simulink model "state_space_simulink_feedback_control101"  (R2023b)
settings: Solver=VariableStepAuto  StartTime=0.0  StopTime=endtime  RelTol=1e-3
undefined symbols (not defined in the file or in its folder): A, B, C, Cx, Dx, K, x0
settings Model: Creator=Anthony  LastModifiedBy=Anthony Rossiter
settings DataIOCC: SaveFormat=Structure  SignalLogging=off
settings ModelReferenceCC: EnableRefExpFcnMdlSchedulingChecks=on

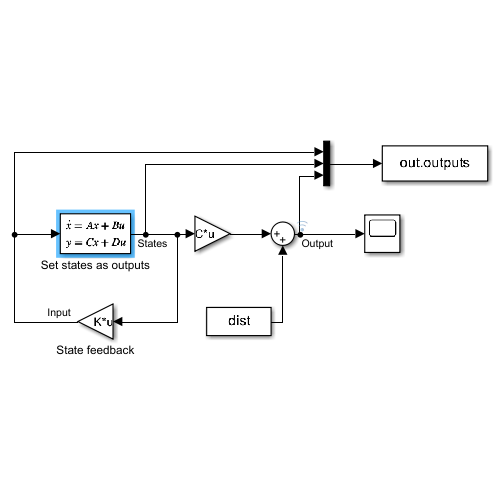
[thumbnail: Simulink's stored preview of the top-level diagram]
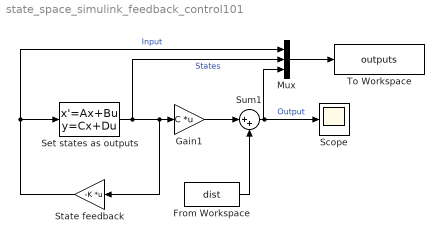
== system state_space_simulink_feedback_control101 ==
  From Workspace : FromWorkspace  VariableName=dist
  Gain1 : Gain  Gain=C  Multiplication=Matrix(K*u)
  Mux : Mux  Inputs=3
  Scope : Scope
  Set states as outputs : StateSpace  A=A  B=B  C=Cx  D=Dx  InitialCondition=x0
  State feedback : Gain  Gain=-K  Multiplication=Matrix(K*u)
  Sum1 : Sum  Inputs=|++
  To Workspace : ToWorkspace  VariableName=outputs  SaveFormat=Structure With Time  SampleTime=-1
  wires:
  Set states as outputs/1 -> Mux/2, Gain1/1, State feedback/1  "States"
  Gain1/1 -> Sum1/1
  Sum1/1 -> Scope/1, Mux/3  "Output"
  From Workspace/1 -> Sum1/2
  State feedback/1 -> Mux/1, Set states as outputs/1  "Input"
  Mux/1 -> To Workspace/1
